simulink model "X1PFjicheng"  (R2024a)
settings: Solver=ode4  StartTime=0.0  StopTime=inf  FixedStep=0.05  RelTol=1e-3
values from neighbouring files (symbols this model uses):
  A0 = [app.A0XEditField.Value, app.A0YEditField.Value, app.A0ZEditField.Value]    [sendDubinsTCPData.m]    (also in sendLocalTCPData.m; sendTCPData.m)
  Delta = [app.Delta1EditField.Value,app.Delta2EditField.Value,app.Delta3EditField.Value,app.Delta4EditField.Value]    [sendDubinsTCPData.m]    (also in sendTCPData.m)
  down = app.downEditField.Value    [sendDubinsTCPData.m]    (also in sendTCPData.m)
  Kdelta = [app.Kdelta1EditField.Value,app.Kdelta2EditField.Value,app.Kdelta3EditField.Value,app.Kdelta4EditField.Value]    [sendDubinsTCPData.m]    (also in sendTCPData.m)
  P0 = [app.P0XEditField.Value, app.P0YEditField.Value, app.P0ZEditField.Value]    [sendDubinsTCPData.m]    (also in sendLocalTCPData.m; sendTCPData.m)
  Td = app.TdEditField.Value    [sendDubinsTCPData.m]    (also in sendTCPData.m)
  Tj = app.TjEditField.Value    [sendDubinsTCPData.m]    (also in sendTCPData.m)
  ud = app.udEditField.Value    [sendDubinsTCPData.m]    (also in sendTCPData.m)
  up = app.upEditField.Value    [sendDubinsTCPData.m]    (also in sendTCPData.m)
  Waypoints = evalin('base', 'Waypoints')    [planAUVPaths.m]    (also in planUAVPaths.m = csvread('CSV_waypoints.csv', 1, 0); sendTCPData.m = [app.Waypoints, column_of_z])
  WPNum = size(result_no_duplicates, 1)    [sendDubinsTCPData.m]    (also in sendLocalTCPData.m = size(waypoints, 1); sendTCPData.m = size(app.Waypoints, 1))
  z = app.ZEditField.Value    [sendDubinsTCPData.m]    (also in sendTCPData.m)
libraries: slpidlib x2
(part 1 of 2)
settings Model: Creator=22979  LastModifiedBy=22979
settings DataIOCC: SaveOperatingPoint=on  InspectSignalLogs=on  ReturnWorkspaceOutputs=off  LoggingFileName=losout.mat
settings DebuggingCC: AlgebraicLoopMsg=none  UnconnectedInputMsg=warning  UnconnectedOutputMsg=warning  UnconnectedLineMsg=warning
settings ModelReferenceCC: EnableRefExpFcnMdlSchedulingChecks=on
settings RTWCC: PackageGeneratedCodeAndArtifacts=on  GPUComputeCapability=3.5  DLArmComputeVersion=19.05

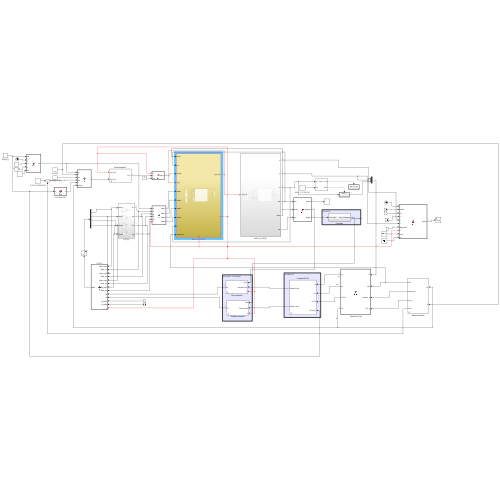
[thumbnail: Simulink's stored preview of the top-level diagram]
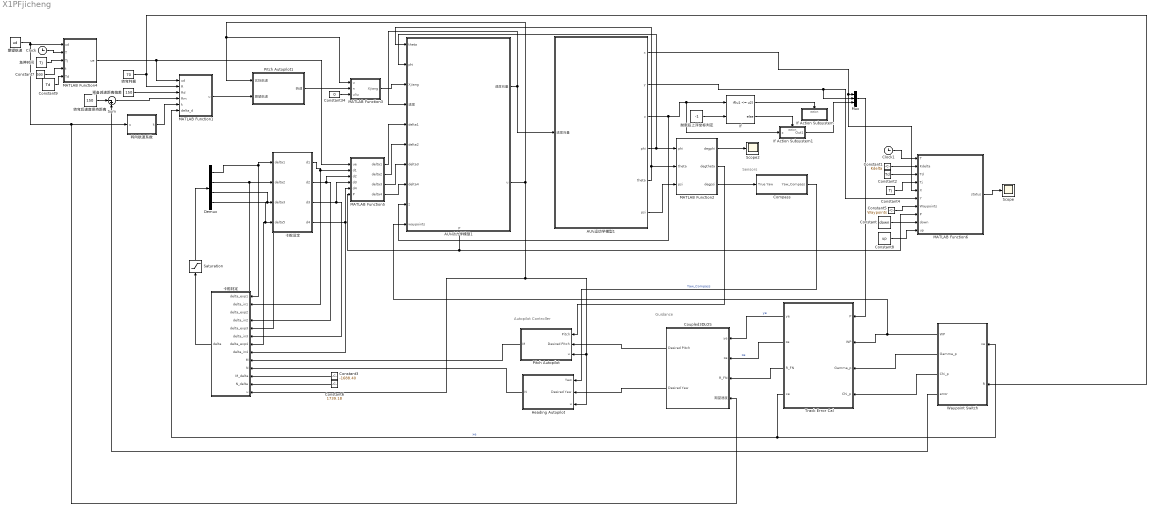
== system X1PFjicheng ==
  note: Sensors
  note: Guidance
  note: Autopilot Controller
  AUV动力学模型1 : Subsystem
      settings: PortSchema="{\"entries\":[{\"content\":{\"sides\":[{\"content\":{\"connectorIds\":[\"In1\",\"In2\",\"In3\",\"In4\",\"In5\",\"In6\",\"In7\",\"In8\",\"In9\",\"In10\"]},\"type\":\"ConnectorPlacement.EquallySpacedRectSide\",\"uuid\":\"1654708e-3081-4ea6-965b-5b7cd41b3ec5\"},{\"content\":{\"connectorIds\":[\"Out1\",\"Out2\"],\"side\":\"RIGHT\"},\"type\":\"ConnectorPlacement.EquallySpacedRectSide\",\"uuid\":\"9e07aa6c-7bc5-448a-bff9-c01bf6300cbd\"},{\"content\":{\"side\":\"TOP\"},\"type\":\"ConnectorPlacement.EquallySpacedRectSide\",\"uuid\":\"c074f735-85a1-4ba5-b9fb-1975a738e7a6\"},{\"content\":{\"connectorIds\":[\"Out3\"],\"side\":\"BOTTOM\"},\"type\":\"ConnectorPlacement.EquallySpacedRectSide\",\"uuid\":\"ec244679-bb4c-412e-b3fb-81b5c85a18e4\"}]},\"type\":\"ConnectorPlacement.EquallySpacedConnector\",\"uuid\":\"11f0b0be-650c-4135-b043-c000e16f372f\"}],\"packageUris\":[\"http://schema.mathworks.com/mf0/Connector/R2020b\"],\"version\":\"1.0\"}"
  AUV运动学模型1 : Subsystem
  Clock : Clock
  Clock1 : Clock
  Compass : Subsystem
  Constant : Constant  Value=down
  Constant1 : Constant  Value=Kdelta
  Constant2 : Constant  Value=Td
  Constant3 : Constant  Value=-1688.40
  Constant34 : Constant  Value=0
  Constant4 : Constant  Value=Tj
  Constant5 : Constant  Value=Waypoints
  Constant6 : Constant  Value=1739.18
  Constant7 : Constant  Value=500
  Constant8 : Constant  Value=up
  Constant9 : Constant  Value=Td
  Coupled3DLOS : Subsystem  mask{LOSAlg=LOS, Delta=26, Kapa=0.25, Gamma=0.3}
      mask prompts: LOSAlg "制导算法"; Delta "前视距离"; Kapa "漂角自适应估计增益"; Gamma "攻角自适应估计增益"
      mask TypeOptions LOSAlg: LOS | ALOS
      mask DialogControl DescGroupVar Prompt: 三维视线角制导
      mask DialogControl DescTextVar Prompt: 设置三维视线角制导参数：前视距离，漂角自适应估计增益，漂角自适应估计增益。自适应估计增益设置为0，屏蔽估计补偿；非0，启用估计补偿。
      mask DialogControl Container5 Prompt: 旋转制导算法
      mask DialogControl ParameterGroupVar Prompt: 设置制导参数
  Demux : Demux
  Heading Autopilot : Subsystem  mask{kp=1500, ki=0, kd=500}
      mask DialogControl DescGroupVar Prompt: Heading Autopilot
      mask DialogControl DescTextVar Prompt: 设置PID增益。
      mask DialogControl ParameterGroupVar Prompt: PID Parameter
  If : If  NumInputs=2  IfExpression=u1 <= u2
  If Action Subsystem : Subsystem  TreatAsAtomicUnit=on
  If Action Subsystem1 : Subsystem  TreatAsAtomicUnit=on
  MATLAB Function1 : MATLAB Function  TreatAsAtomicUnit=on
  MATLAB Function2 : MATLAB Function  TreatAsAtomicUnit=on
  MATLAB Function3 : MATLAB Function  TreatAsAtomicUnit=on
  MATLAB Function4 : MATLAB Function  TreatAsAtomicUnit=on
  MATLAB Function5 : MATLAB Function  TreatAsAtomicUnit=on
  MATLAB Function6 : MATLAB Function  TreatAsAtomicUnit=on
  Mux : Mux  Inputs=3
  Pitch Autopilot : Subsystem  mask{kp=2400, ki=0, kd=500}
      mask DialogControl DescGroupVar Prompt: Pitch Autopilot
      mask DialogControl DescTextVar Prompt: 设置PID控制增益。
      mask DialogControl ParameterGroupVar Prompt: PID Parameter
  Pitch Autopilot1 : Subsystem  mask{kp=600, ki=20, kd=0}
      mask DialogControl DescGroupVar Prompt: Pitch Autopilot
      mask DialogControl DescTextVar Prompt: 设置PID控制增益。
      mask DialogControl ParameterGroupVar Prompt: PID Parameter
  Saturation : Saturate  UpperLimit=0.4363  LowerLimit=-0.4363
  Scope : Scope
  Scope2 : Scope
  Sum : Sum  Inputs=|-+
  Track Error Cal : MATLAB Function  TreatAsAtomicUnit=on
  Waypoint Switch : Subsystem  mask{WP=Waypoints, WPNum=WPNum}
      mask prompts: WP "航点序列"; WPNum "航点个数"
      mask DialogControl DescGroupVar Prompt: 航点设置
      mask DialogControl DescTextVar Prompt: 设置航点序列和个数
  卡舵判定 : MATLAB Function  TreatAsAtomicUnit=on
  卡舵设定 : Subsystem
  急停时间 : Constant  Value=Tj
  抛载后上浮坐标判定 : Constant  Value=-1
  期望航速 : Constant  Value=ud
  转向航速系数 : MATLAB Function  TreatAsAtomicUnit=on
  转弯判据 : Constant  Value=70
  转弯后速度保持距离 : Constant  Value=150
  预备减速距离偏差 : Constant  Value=150
  wires:
  AUV运动学模型1/1(x) -> MATLAB Function6/5(X), Mux/1
  AUV运动学模型1/3(z) -> If/1, If Action Subsystem1/1(z), AUV动力学模型1/9(z)
  AUV运动学模型1/4(phi) -> MATLAB Function2/1(phi), AUV动力学模型1/2(phi)
  AUV运动学模型1/5(theta) -> AUV动力学模型1/1(theta), MATLAB Function2/2(theta)
  AUV运动学模型1/6(psi) -> MATLAB Function2/3(psi)
  AUV动力学模型1/1(速度向量) -> AUV动力学模型1/4(速度), AUV运动学模型1/1(速度向量)
  Track Error Cal/4(xe) -> Waypoint Switch/1(xe), MATLAB Function1/6(delta_d)  "xe"
  Waypoint Switch/3(Chi_p) -> Track Error Cal/4(Chi_p)
  Waypoint Switch/1(WP) -> AUV动力学模型1/10(waypoints), Track Error Cal/2(WP)
  Track Error Cal/2(ze) -> Coupled3DLOS/2(ze)  "ze"
  Track Error Cal/1(ye) -> Coupled3DLOS/1(ye)  "ye"
  Waypoint Switch/2(Gamma_p) -> Track Error Cal/3(Gamma_p)
  Track Error Cal/3(R_FN) -> Coupled3DLOS/3(R_FN)
  Coupled3DLOS/1(Desired Pitch) -> Pitch Autopilot/2(Desired Pitch)
  Coupled3DLOS/2(Desired Yaw) -> Heading Autopilot/2(Desired Yaw)
  Compass/1(Yaw_Compass) -> Heading Autopilot/1(Yaw)  "Yaw_Compass"
  MATLAB Function1/1(u) -> Pitch Autopilot1/2(期望航速)
  转弯后速度保持距离/1 -> Sum/1
  Pitch Autopilot1/1(转速) -> MATLAB Function3/2(n)
  Sum/1 -> MATLAB Function1/4(Rm)
  Constant34/1 -> MATLAB Function3/3(uliu)
  预备减速距离偏差/1 -> MATLAB Function1/3(Rd)
  转弯判据/1 -> Waypoint Switch/2(R), MATLAB Function1/2(R)
  AUV动力学模型1/2(u) -> Pitch Autopilot1/1(实际航速), MATLAB Function3/1(u), 卡舵判定/13(u), Pitch Autopilot/3(u), Heading Autopilot/3(u)
  Waypoint Switch/4(error) -> Sum/2
  AUV运动学模型1/2(y) -> Mux/2, MATLAB Function6/6(Y)
  Mux/1 -> Track Error Cal/1(P)
  MATLAB Function3/1(Xjiang) -> AUV动力学模型1/3(Xjiang)
  MATLAB Function2/2(degtheta) -> Pitch Autopilot/1(Pitch)
  MATLAB Function2/3(degpsi) -> Compass/1(True Yaw)
  Saturation/1 -> Demux/1
  MATLAB Function2/1(degphi) -> Scope2/1
  Demux/1 -> 卡舵判定/1(delta_exp1), 卡舵设定/1(delta1)
  卡舵设定/4(d4) -> MATLAB Function5/5(d4), 卡舵判定/8(delta_in4)
  Demux/2 -> 卡舵判定/3(delta_exp2), 卡舵设定/2(delta2)
  Demux/4 -> 卡舵设定/4(delta5), 卡舵判定/7(delta_exp4)
  Pitch Autopilot/1(M) -> 卡舵判定/9(M)
  Heading Autopilot/1(N) -> 卡舵判定/10(N)
  Constant3/1 -> 卡舵判定/11(M_delta)
  Constant6/1 -> 卡舵判定/12(N_delta)
  卡舵判定/1(delta) -> Saturation/1
  Demux/3 -> 卡舵判定/5(delta_exp3), 卡舵设定/3(delta3)
  卡舵设定/1(d1) -> 卡舵判定/2(delta_in1), MATLAB Function5/2(d1)
  卡舵设定/2(d2) -> MATLAB Function5/3(d2), 卡舵判定/4(delta_in2)
  卡舵设定/3(d3) -> MATLAB Function5/4(d3), 卡舵判定/6(delta_in3)
  抛载后上浮坐标判定/1 -> If/2
  If/1 -> If Action Subsystem/Action
  If/2 -> If Action Subsystem1/Action
  If Action Subsystem1/1(Out1) -> Mux/3
  Clock/1 -> MATLAB Function4/2(T)
  期望航速/1 -> Coupled3DLOS/4(期望速度), 转向航速系数/1(u), MATLAB Function4/1(ud)
  急停时间/1 -> MATLAB Function4/3(Tj)
  AUV动力学模型1/3(P) -> MATLAB Function5/6(P), MATLAB Function6/8(P)
  MATLAB Function5/1(delta1) -> AUV动力学模型1/5(delta1)
  MATLAB Function5/2(delta2) -> AUV动力学模型1/6(delta2)
  MATLAB Function5/3(delta3) -> AUV动力学模型1/7(delta3)
  MATLAB Function5/4(delta4) -> AUV动力学模型1/8(delta4)
  Constant1/1 -> MATLAB Function6/2(Kdelta)
  Constant2/1 -> MATLAB Function6/3(Td)
  Constant4/1 -> MATLAB Function6/4(Tj)
  MATLAB Function6/1(status) -> Scope/1
  Clock1/1 -> MATLAB Function6/1(T)
  Constant5/1 -> MATLAB Function6/7(Waypoints)
  Constant7/1 -> MATLAB Function4/4(t)
  MATLAB Function4/1(ue) -> MATLAB Function5/1(ue), MATLAB Function1/1(ud)
  转向航速系数/1(k) -> MATLAB Function1/5(k)
  Constant/1 -> MATLAB Function6/9(down)
  Constant8/1 -> MATLAB Function6/10(up)
  Constant9/1 -> MATLAB Function4/5(Td)

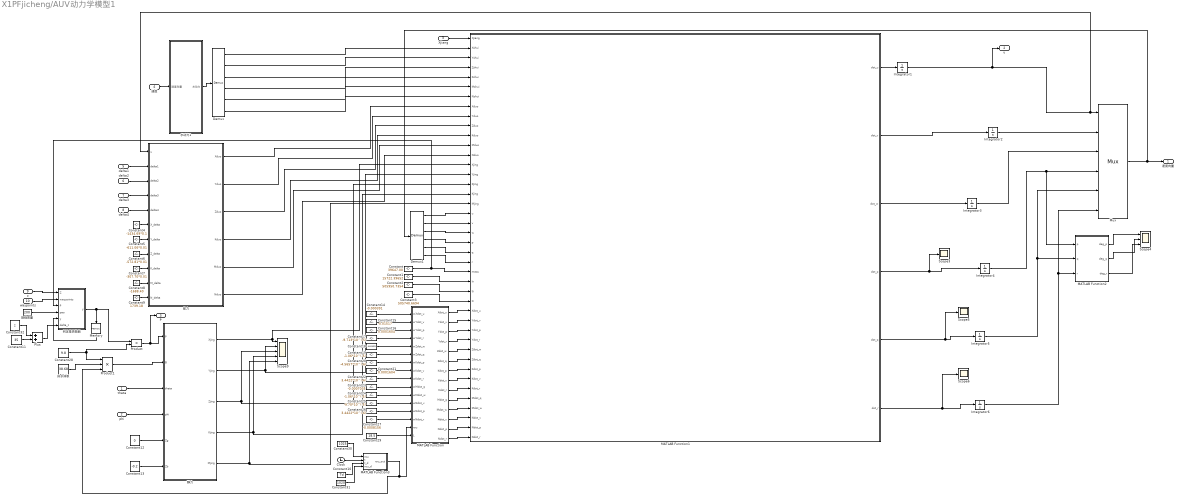
== system X1PFjicheng/AUV动力学模型1 ==
  theta : Inport
  phi : Inport  Port=2
  Xjiang : Inport  Port=3
  速度 : Inport  Port=4
  delta1 : Inport  Port=5
  delta2 : Inport  Port=6
  delta3 : Inport  Port=7
  delta4 : Inport  Port=8
  z : Inport  Port=9
  waypoints : Inport  Port=10
  Clock : Clock
  Constant : Constant  Value=39647.00
  Constant1 : Constant  Value=15722.39652
  Constant10 : Constant  Value=Td
  Constant11 : Constant  Value=35
  Constant12 : Constant  Value=0
  Constant13 : Constant  Value=-0.2
  Constant14 : Constant  Value=-0.000391
  Constant15 : Constant  Value=-0.01517
  Constant16 : Constant  Value=0.0001604
  Constant17 : Constant  Value=-9.713*10^(-5)
  Constant18 : Constant  Value=-0.0113
  Constant19 : Constant  Value=-1.06*10^(-5)
  Constant2 : Constant  Value=505950.7354
  Constant20 : Constant  Value=-4.5657*10^(-6)
  Constant21 : Constant  Value=0.0001604
  Constant22 : Constant  Value=3.4422*10^(-6)
  Constant23 : Constant  Value=-0.0007035
  Constant24 : Constant  Value=-1.06*10^(-5)
  Constant25 : Constant  Value=-9.70*10^(-5)
  Constant26 : Constant  Value=3.4422*10^(-6)
  Constant27 : Constant  Value=-0.0008156
  Constant28 : Constant  Value=9.8
  Constant29 : Constant  Value=18.5
  Constant3 : Constant  Value=505740.6694
  Constant30 : Constant  Value=1025
  Constant31 : Constant  Value=1020
  Constant32 : Constant  Value=z
  Constant4 : Constant  Value=-1434.69*0.1
  Constant5 : Constant  Value=-611.06*0.01
  Constant6 : Constant  Value=-572.81*0.01
  Constant7 : Constant  Value=-307.70*0.01
  Constant8 : Constant  Value=-1688.40
  Constant9 : Constant  Value=1739.18
  Demux : Demux  Outputs=6
  Demux1 : Demux  Outputs=6
  Integrator1 : Integrator  InitialCondition=0.01
  Integrator{2..6} (5 alike) : Integrator
  MATLAB Function : MATLAB Function  TreatAsAtomicUnit=on
  MATLAB Function1 : MATLAB Function  TreatAsAtomicUnit=on
  MATLAB Function2 : MATLAB Function  TreatAsAtomicUnit=on
  MATLAB Function3 : MATLAB Function  TreatAsAtomicUnit=on
  Memory : Memory
  Mux : Mux  Inputs=6
  Plus : Sum
  Product : Product
  Product1 : Product  Inputs=3
  Scope3 : Scope
  Scope4 : Scope  NumInputPorts=3
  Scope5 : Scope
  Scope6 : Scope
  Scope9 : Scope  NumInputPorts=5
  判定是否抛载 : MATLAB Function  TreatAsAtomicUnit=on
      settings: MinAlgLoopOccurrences=on
  抛载质量 : Constant  Value=200
  排水体积 : Constant  Value=38.68
  水动力1 : Subsystem
  舵力 : MATLAB Function  TreatAsAtomicUnit=on
  静力 : MATLAB Function  TreatAsAtomicUnit=on
  速度向量 : Outport
  u : Outport  Port=2
  P : Outport  Port=3
  wires:
  Integrator2/1 -> Mux/2
  Integrator5/1 -> MATLAB Function2/2(q), Mux/5
  Integrator3/1 -> Mux/3
  Integrator4/1 -> MATLAB Function2/1(p), Mux/4
  Integrator6/1 -> MATLAB Function2/3(r), Mux/6
  MATLAB Function1/3(dot_w) -> Integrator3/1
  MATLAB Function1/4(dot_p) -> Scope3/1, Integrator4/1
  MATLAB Function1/5(dot_q) -> Scope5/1, Integrator5/1
  MATLAB Function1/6(dot_r) -> Scope6/1, Integrator6/1
  MATLAB Function1/1(dot_u) -> Integrator1/1
  theta/1 -> 静力/3(theta)
  Mux/1 -> 速度向量/1, Demux1/1
  Demux/1 -> MATLAB Function1/2(Xshui)
  Demux/2 -> MATLAB Function1/3(Yshui)
  Demux/3 -> MATLAB Function1/4(Zshui)
  Demux/4 -> MATLAB Function1/5(Kshui)
  Demux/5 -> MATLAB Function1/6(Mshui)
  Demux/6 -> MATLAB Function1/7(Nshui)
  舵力/1(Xduo) -> MATLAB Function1/8(Xduo)
  舵力/2(Yduo) -> MATLAB Function1/9(Yduo)
  舵力/3(Zduo) -> MATLAB Function1/10(Zduo)
  舵力/4(Kduo) -> MATLAB Function1/11(Kduo)
  舵力/5(Mduo) -> MATLAB Function1/12(Mduo)
  舵力/6(Nduo) -> MATLAB Function1/13(Nduo)
  静力/1(Xjing) -> Scope9/1, MATLAB Function1/14(Xjing)
  静力/2(Yjing) -> MATLAB Function1/15(Yjing), Scope9/2
  静力/3(Zjing) -> MATLAB Function1/16(Zjing), Scope9/3
  静力/4(Kjing) -> MATLAB Function1/17(Kjing), Scope9/4
  静力/5(Mjing) -> MATLAB Function1/18(Mjing), Scope9/5
  Demux1/2 -> MATLAB Function1/20(v)
  Demux1/3 -> MATLAB Function1/21(w)
  Demux1/4 -> MATLAB Function1/22(p)
  Demux1/5 -> MATLAB Function1/23(q)
  Demux1/6 -> MATLAB Function1/24(r)
  Constant3/1 -> MATLAB Function1/28(Iz)
  Demux1/1 -> MATLAB Function1/19(u)
  Constant/1 -> 判定是否抛载/3(P), MATLAB Function1/25(mass)
  phi/1 -> 静力/4(phi)
  Constant12/1 -> 静力/5(Zg)
  Constant13/1 -> 静力/6(Zb)
  Constant2/1 -> MATLAB Function1/27(Iy)
  Constant1/1 -> MATLAB Function1/26(Ix)
  Constant14/1 -> MATLAB Function/1(wXdot_u)
  MATLAB Function/1(Xdot_u) -> MATLAB Function1/29(Xdot_u)
  MATLAB Function/2(Ydot_v) -> MATLAB Function1/30(Ydot_v)
  MATLAB Function/3(Ydot_p) -> MATLAB Function1/31(Ydot_p)
  MATLAB Function/4(Ydot_r) -> MATLAB Function1/32(Ydot_r)
  MATLAB Function/5(Zdot_w) -> MATLAB Function1/33(Zdot_w)
  MATLAB Function/6(Zdot_q) -> MATLAB Function1/34(Zdot_q)
  MATLAB Function/7(Kdot_p) -> MATLAB Function1/35(Kdot_p)
  MATLAB Function/8(Kdot_v) -> MATLAB Function1/36(Kdot_v)
  MATLAB Function/9(Kdot_r) -> MATLAB Function1/37(Kdot_r)
  MATLAB Function/10(Mdot_q) -> MATLAB Function1/38(Mdot_q)
  MATLAB Function/11(Mdot_w) -> MATLAB Function1/39(Mdot_w)
  MATLAB Function/12(Ndot_v) -> MATLAB Function1/40(Ndot_v)
  MATLAB Function/13(Ndot_p) -> MATLAB Function1/41(Ndot_p)
  MATLAB Function/14(Ndot_r) -> MATLAB Function1/42(Ndot_r)
  Constant15/1 -> MATLAB Function/2(wYdot_v)
  Constant16/1 -> MATLAB Function/3(wYdot_p)
  Constant17/1 -> MATLAB Function/4(wYdot_r)
  Constant18/1 -> MATLAB Function/5(wZdot_w)
  Constant19/1 -> MATLAB Function/6(wZdot_q)
  Constant20/1 -> MATLAB Function/7(wKdot_p)
  Constant21/1 -> MATLAB Function/8(wKdot_v)
  Constant22/1 -> MATLAB Function/9(wKdot_r)
  Constant23/1 -> MATLAB Function/10(wMdot_q)
  Constant24/1 -> MATLAB Function/11(wMdot_w)
  Constant25/1 -> MATLAB Function/12(wNdot_v)
  Constant26/1 -> MATLAB Function/13(wNdot_p)
  Constant27/1 -> MATLAB Function/14(wNdot_r)
  Constant29/1 -> MATLAB Function/16(L)
  Integrator1/1 -> u/1, Mux/1, 舵力/1(u)
  MATLAB Function1/2(dot_v) -> Integrator2/1
  MATLAB Function2/1(deg_p) -> Scope4/1
  MATLAB Function2/2(deg_q) -> Scope4/2
  MATLAB Function2/3(deg_r) -> Scope4/3
  Constant4/1 -> 舵力/6(X_delta)
  Constant6/1 -> 舵力/8(Z_delta)
  Constant7/1 -> 舵力/9(K_delta)
  Constant8/1 -> 舵力/10(M_delta)
  Constant9/1 -> 舵力/11(N_delta)
  Constant5/1 -> 舵力/7(Y_delta)
  水动力1/1(水动力) -> Demux/1
  速度/1 -> 水动力1/1(速度向量)
  Xjiang/1 -> MATLAB Function1/1(Xjiang)
  Clock/1 -> MATLAB Function3/2(t)
  Constant30/1 -> MATLAB Function3/1(rou)
  MATLAB Function3/1(rou_out) -> Product1/3, MATLAB Function/15(rou)
  排水体积/1 -> Product1/2
  Constant28/1 -> Product/2, Product1/1
  Product1/1 -> 静力/2(B)
  Constant31/1 -> MATLAB Function3/4(rou_d)
  Constant10/1 -> MATLAB Function3/3(t_d)
  抛载质量/1 -> 判定是否抛载/4(pao)
  waypoints/1 -> 判定是否抛载/2(waypoints)
  z/1 -> 判定是否抛载/1(Z)
  Product/1 -> P/1, 静力/1(P)
  判定是否抛载/1(y) -> Memory/1, Product/1
  Memory/1 -> 判定是否抛载/5("y ")
  delta1/1 -> 舵力/2(delta1)
  delta2/1 -> 舵力/3(delta2)
  delta3/1 -> 舵力/4(delta3)
  delta4/1 -> 舵力/5(delta4)
  Constant11/1 -> Plus/2
  Plus/1 -> 判定是否抛载/6(delta_z)
  Constant32/1 -> Plus/1

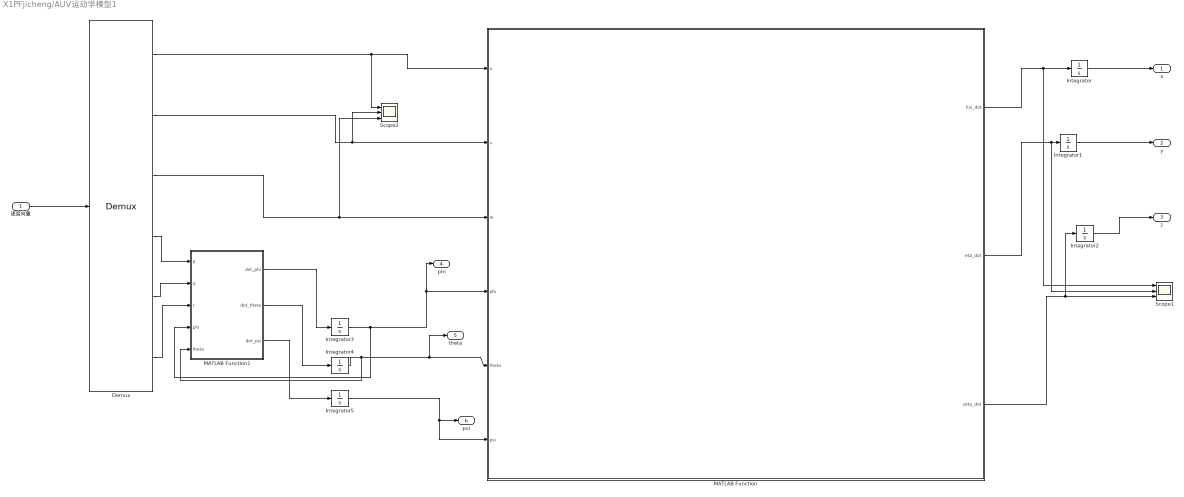
== system X1PFjicheng/AUV运动学模型1 ==
  速度向量 : Inport
  Demux : Demux  Outputs=6
  Integrator : Integrator  InitialCondition=P0(1)
  Integrator1 : Integrator  InitialCondition=P0(2)
  Integrator2 : Integrator  InitialCondition=P0(3)
  Integrator3 : Integrator  InitialCondition=A0(1)*pi/180
  Integrator4 : Integrator  InitialCondition=A0(2)*pi/180
  Integrator5 : Integrator  InitialCondition=A0(3)*pi/180
  MATLAB Function : MATLAB Function  TreatAsAtomicUnit=on
  MATLAB Function1 : MATLAB Function  TreatAsAtomicUnit=on
  Scope1 : Scope  NumInputPorts=3
  Scope2 : Scope  NumInputPorts=3
  x : Outport
  y : Outport  Port=2
  z : Outport  Port=3
  phi : Outport  Port=4
  theta : Outport  Port=5
  psi : Outport  Port=6
  wires:
  Integrator2/1 -> z/1
  Integrator1/1 -> y/1
  MATLAB Function/2(eta_dot) -> Scope1/2, Integrator1/1
  MATLAB Function/1(ksi_dot) -> Integrator/1, Scope1/1
  MATLAB Function/3(zeta_dot) -> Integrator2/1, Scope1/3
  Demux/1 -> Scope2/1, MATLAB Function/1(u)
  Demux/2 -> Scope2/2, MATLAB Function/2(v)
  Demux/3 -> Scope2/3, MATLAB Function/3(w)
  速度向量/1 -> Demux/1
  Integrator3/1 -> MATLAB Function1/4(phi), MATLAB Function/4(phi), phi/1
  Integrator4/1 -> MATLAB Function1/5(theta), theta/1, MATLAB Function/5(theta)
  Integrator5/1 -> MATLAB Function/6(psi), psi/1
  Demux/5 -> MATLAB Function1/2(q)
  Demux/4 -> MATLAB Function1/1(p)
  Demux/6 -> MATLAB Function1/3(r)
  MATLAB Function1/1(dot_phi) -> Integrator3/1
  MATLAB Function1/2(dot_theta) -> Integrator4/1
  MATLAB Function1/3(dot_psi) -> Integrator5/1
  Integrator/1 -> x/1

== system X1PFjicheng/Compass ==
  True Yaw : Inport
  Add : Sum
  Add1 : Sum
  Add2 : Sum
  Constant : Constant  Value=round(rand*20-10)
  Constant1 : Constant  Value=0
  Gain : Gain  Gain=0
  Integrator : Integrator
  MATLAB Function : MATLAB Function  TreatAsAtomicUnit=on
  Random Number : RandomNumber  Commented=on  Variance=0.05  Seed=round(rand*20)  SampleTime=1
  Yaw_Compass : Outport
  wires:
  Constant/1 -> Add1/2  "bias"
  Integrator/1 -> Add1/1, Gain/1  "noise"
  Gain/1 -> Add/2
  Add/1 -> Integrator/1
  Add1/1 -> Add2/1  "Compass_Noise"
  True Yaw/1 -> Add2/2
  MATLAB Function/1(u) -> Yaw_Compass/1
  Add2/1 -> MATLAB Function/1(in)
  Constant1/1 -> Add/1

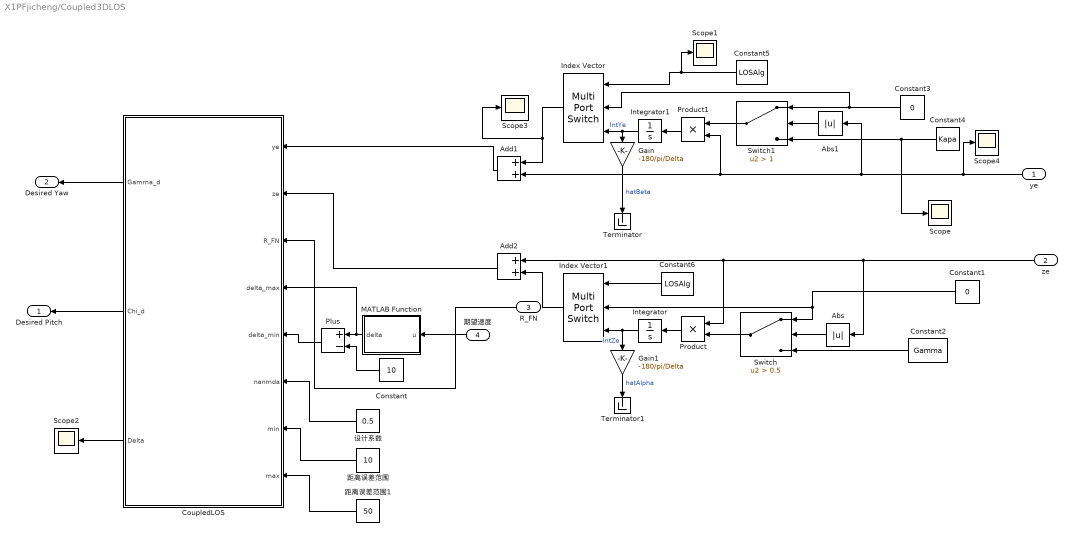
== system X1PFjicheng/Coupled3DLOS ==
  ye : Inport
  ze : Inport  Port=2
  R_FN : Inport  Port=3
  期望速度 : Inport  Port=4
  Abs : Abs  SaturateOnIntegerOverflow=off
  Abs1 : Abs  SaturateOnIntegerOverflow=off
  Add1 : Sum
  Add2 : Sum
  Constant : Constant  Value=10
  Constant1 : Constant  Value=0
  Constant2 : Constant  Value=Gamma
  Constant3 : Constant  Value=0
  Constant4 : Constant  Value=Kapa
  Constant5 : Constant  Value=LOSAlg
  Constant6 : Constant  Value=LOSAlg
  CoupledLOS : MATLAB Function  TreatAsAtomicUnit=on
  Gain : Gain  Gain=-180/pi/Delta
  Gain1 : Gain  Gain=-180/pi/Delta
  Index Vector : MultiPortSwitch  Inputs=2  SaturateOnIntegerOverflow=off  InputSameDT=off
  Index Vector1 : MultiPortSwitch  Inputs=2  SaturateOnIntegerOverflow=off  InputSameDT=off
  Integrator : Integrator
  Integrator1 : Integrator
  MATLAB Function : MATLAB Function  TreatAsAtomicUnit=on
  Plus : Sum  Inputs=+-
  Product : Product
  Product1 : Product
  Scope{,1..4} (5 alike) : Scope
  Switch : Switch  Criteria=u2 > Threshold  Threshold=0.5  SaturateOnIntegerOverflow=off  InputSameDT=off
  Switch1 : Switch  Criteria=u2 > Threshold  Threshold=1  SaturateOnIntegerOverflow=off  InputSameDT=off
  Terminator : Terminator
  Terminator1 : Terminator
  设计系数 : Constant  Value=0.5
  距离误差范围 : Constant  Value=10
  距离误差范围1 : Constant  Value=50
  Desired Pitch : Outport
  Desired Yaw : Outport  Port=2
  wires:
  Abs1/1 -> Switch1/2
  ze/1 -> Abs/1, Add2/1, Product/1
  Constant2/1 -> Switch/3
  Abs/1 -> Switch/2
  Product/1 -> Integrator/1
  Constant4/1 -> Scope/1, Switch1/3
  Constant1/1 -> Index Vector1/2, Switch/1
  ye/1 -> Add1/2, Product1/2, Abs1/1, Scope4/1
  Integrator/1 -> Gain1/1, Index Vector1/3  "IntZe"
  Add2/1 -> CoupledLOS/2(ze)
  Product1/1 -> Integrator1/1
  Switch/1 -> Product/2
  CoupledLOS/2(Chi_d) -> Desired Pitch/1
  Switch1/1 -> Product1/1
  Constant3/1 -> Index Vector/2, Switch1/1
  Add1/1 -> CoupledLOS/1(ye)
  CoupledLOS/1(Gamma_d) -> Desired Yaw/1
  Integrator1/1 -> Gain/1, Index Vector/3  "IntYe"
  R_FN/1 -> CoupledLOS/3(R_FN)
  Constant5/1 -> Scope1/1, Index Vector/1
  Index Vector/1 -> Add1/1, Scope3/1
  Constant6/1 -> Index Vector1/1
  Index Vector1/1 -> Add2/2
  Gain/1 -> Terminator/1  "hatBeta"
  Gain1/1 -> Terminator1/1  "hatAlpha"
  MATLAB Function/1(delta) -> CoupledLOS/4(delta_max), Plus/1
  设计系数/1 -> CoupledLOS/6(nanmda)
  距离误差范围/1 -> CoupledLOS/7(min)
  距离误差范围1/1 -> CoupledLOS/8(max)
  CoupledLOS/3(Delta) -> Scope2/1
  期望速度/1 -> MATLAB Function/1(u)
  Plus/1 -> CoupledLOS/5(delta_min)
  Constant/1 -> Plus/2

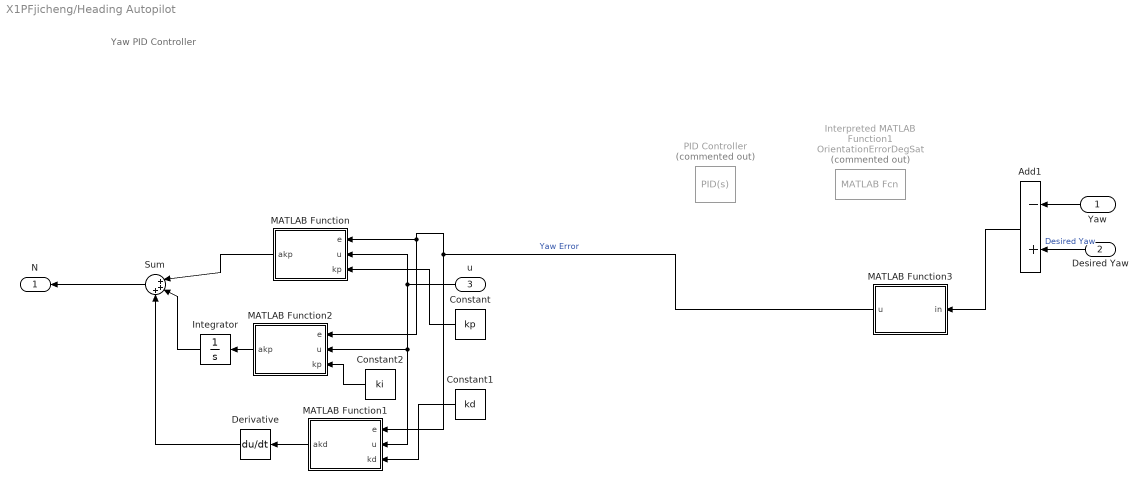
== system X1PFjicheng/Heading Autopilot ==
  note: Yaw PID Controller
  Yaw : Inport
  Desired Yaw : Inport  Port=2
  u : Inport  Port=3
  Add1 : Sum  Inputs=-+
  Constant : Constant  Value=kp
  Constant1 : Constant  Value=kd
  Constant2 : Constant  Value=ki
  Derivative : Derivative
  Integrator : Integrator
  Interpreted MATLAB Function1 : MATLABFcn  Commented=on  MATLABFcn=OrientationErrorDegSat  OutputDimensions=1
  MATLAB Function : MATLAB Function  TreatAsAtomicUnit=on
  MATLAB Function1 : MATLAB Function  TreatAsAtomicUnit=on
  MATLAB Function2 : MATLAB Function  TreatAsAtomicUnit=on
  MATLAB Function3 : MATLAB Function  TreatAsAtomicUnit=on
  PID Controller : slpidlib/PID Controller  Commented=on  Controller=PID  Form=Parallel  TimeDomain=Continuous-time  UseExternalTs=off  SampleTime=-1  IntegratorMethod=Forward Euler  FilterMethod=Forward Euler  ControllerParametersSource=internal  P=kp  I=ki  UseKiTs=off  D=kd  UseExternalDerivativeSource=off  N=100  UseFilter=on  TunerSelectOption=Transfer Function Based (PID Tuner App)  InitialConditionSource=internal  InitialConditionForIntegrator=0  InitialConditionForFilter=0  DifferentiatorICPrevScaledInput=0  ExternalReset=none  TrackingMode=off  Kt=1  LimitOutput=off  SatLimitsSource=internal  UpperSaturationLimit=inf  LowerSaturationLimit=-inf  LinearizeAsGain=on  AntiWindupMode=none  Kb=1  LimitIntegrator=off  UpperIntegratorSaturationLimit=inf  LowerIntegratorSaturationLimit=-inf  POutMin=[]  POutMax=[]  IOutMin=[]  IOutMax=[]  DOutMin=[]  DOutMax=[]  NOutMin=[]  NOutMax=[]  SumOutMin=[]  SumOutMax=[]  SaturationOutMin=[]  SaturationOutMax=[]  PParamMin=[]  PParamMax=[]  IParamMin=[]  IParamMax=[]  DParamMin=[]  DParamMax=[]  NParamMin=[]  NParamMax=[]  KbParamMin=[]  KbParamMax=[]  KtParamMin=[]  KtParamMax=[]  KbOutMin=[]  KbOutMax=[]  KtOutMin=[]  KtOutMax=[]  IntegratorOutMin=[]  IntegratorOutMax=[]  FilterOutMin=[]  FilterOutMax=[]  SumI1OutMin=[]  SumI1OutMax=[]  SumI2OutMin=[]  SumI2OutMax=[]  SumI3OutMin=[]  SumI3OutMax=[]  SumI4OutMin=[]  SumI4OutMax=[]  SumDOutMin=[]  SumDOutMax=[]  DifferentiatorOutMin=[]  DifferentiatorOutMax=[]  FilterDiffOutCoefMin=[]  FilterDiffOutCoefMax=[]  ReciprocalOutMin=[]  ReciprocalOutMax=[]  SumDenOutMin=[]  SumDenOutMax=[]  SumNumOutMin=[]  SumNumOutMax=[]  DivideOutMin=[]  DivideOutMax=[]  UdiffTsProdOutMin=[]  UdiffTsProdOutMax=[]  NTsProdOutMin=[]  NTsProdOutMax=[]  UintegralTsProdOutMin=[]  UintegralTsProdOutMax=[]  UngainTsProdOutMin=[]  UngainTsProdOutMax=[]  ClampingZeroOutDataTypeStr=Inherit: Inherit via back propagation  ClampingZeroOutMin=[]  ClampingZeroOutMax=[]  FilterDenConstantOutDataTypeStr=Inherit: Inherit via back propagation  FilterDenConstantOutMin=[]  FilterDenConstantOutMax=[]  PCopyOutDataTypeStr=Inherit: Inherit via back propagation  PCopyOutMin=[]  PCopyOutMax=[]  NCopyOutDataTypeStr=Inherit: Inherit via back propagation  NCopyOutMin=[]  NCopyOutMax=[]  IntegratorContinuousStateAttributes=''  IntegratorStateMustResolveToSignalObject=off  IntegratorRTWStateStorageClass=Auto  FilterContinuousStateAttributes=''  FilterStateMustResolveToSignalObject=off  FilterRTWStateStorageClass=Auto  ParallelPVariant=InternalParameters  IdealPVariant=Disabled  IVariant=InternalParameters  DVariant=InternalParameters  IntegratorVariant=Continuous  SatVariant=Disabled  AWVariant=Passthrough  PCopyVariant=Disabled  TRVariant=Disabled  FdbkBlocksVariant=Forward  IdealPFdbkVariant=Disabled  SatFdbkVariant=Disabled  DerivativeFilterVariant=ContFilter  NVariant=InternalParameters  NCopyVariant=Disabled  FilterICVariant=InternalICsFilter  IntegratorICVariant=InternalICs  ExternalResetVariant=Disabled  TRSumVariant=Passthrough  SumFdbkVariant=Disabled  SumVariant=Sum_PID  TsampFilterVariant=InternalTs  TsampNgainVariant=Passthrough  TsampIntegralVariant=Disabled_SignalSpec  ExternalSaturationOutDataTypeStr=Inherit: Same as second input  DerivativeSourceVariant=ErrorSignal
  Sum : Sum  Inputs=|+++
  N : Outport
  wires:
  Yaw/1 -> Add1/1
  Add1/1 -> MATLAB Function3/1(in)
  Desired Yaw/1 -> Add1/2  "Desired Yaw"
  Constant1/1 -> MATLAB Function1/3(kd)
  MATLAB Function1/1(akd) -> Derivative/1
  Constant/1 -> MATLAB Function/3(kp)
  u/1 -> MATLAB Function1/2(u), MATLAB Function2/2(u), MATLAB Function/2(u)
  Constant2/1 -> MATLAB Function2/3(kp)
  MATLAB Function2/1(akp) -> Integrator/1
  MATLAB Function/1(akp) -> Sum/1
  Integrator/1 -> Sum/2
  Derivative/1 -> Sum/3
  Sum/1 -> N/1
  MATLAB Function3/1(u) -> MATLAB Function2/1(e), MATLAB Function/1(e), MATLAB Function1/1(e)  "Yaw Error"

== system X1PFjicheng/If Action Subsystem ==
  Action Port : ActionPort  ActionPortLabel=if(u1 <= u2)
  Constant : Constant
  Stop Simulation : Stop
  wires:
  Constant/1 -> Stop Simulation/1

== system X1PFjicheng/If Action Subsystem1 ==
  z : Inport
  Action Port : ActionPort  ActionPortLabel=else
  Out1 : Outport
  wires:
  z/1 -> Out1/1

== system X1PFjicheng/Pitch Autopilot ==
  note: Pitch PID Controller
  Pitch : Inport
  Desired Pitch : Inport  Port=2
  u : Inport  Port=3
  Add1 : Sum  Inputs=-+
  Constant : Constant  Value=kp
  Constant1 : Constant  Value=kd
  Constant2 : Constant  Value=ki
  Derivative : Derivative
  Integrator : Integrator
  MATLAB Function : MATLAB Function  TreatAsAtomicUnit=on
  MATLAB Function1 : MATLAB Function  TreatAsAtomicUnit=on
  MATLAB Function2 : MATLAB Function  TreatAsAtomicUnit=on
  Saturation : Saturate  UpperLimit=25  LowerLimit=-25
  Sum : Sum  Inputs=|+++
  M : Outport
  wires:
  Desired Pitch/1 -> Saturation/1
  Pitch/1 -> Add1/1
  Saturation/1 -> Add1/2  "Desired Pitch"
  Sum/1 -> M/1
  MATLAB Function/1(akp) -> Sum/1
  Constant/1 -> MATLAB Function/3(kp)
  Add1/1 -> MATLAB Function/1(e), MATLAB Function2/1(e), MATLAB Function1/1(e)
  Constant1/1 -> MATLAB Function1/3(kd)
  MATLAB Function1/1(akd) -> Derivative/1
  Derivative/1 -> Sum/2
  u/1 -> MATLAB Function2/2(u), MATLAB Function/2(u), MATLAB Function1/2(u)
  Constant2/1 -> MATLAB Function2/3(ki)
  MATLAB Function2/1(akp) -> Integrator/1
  Integrator/1 -> Sum/3

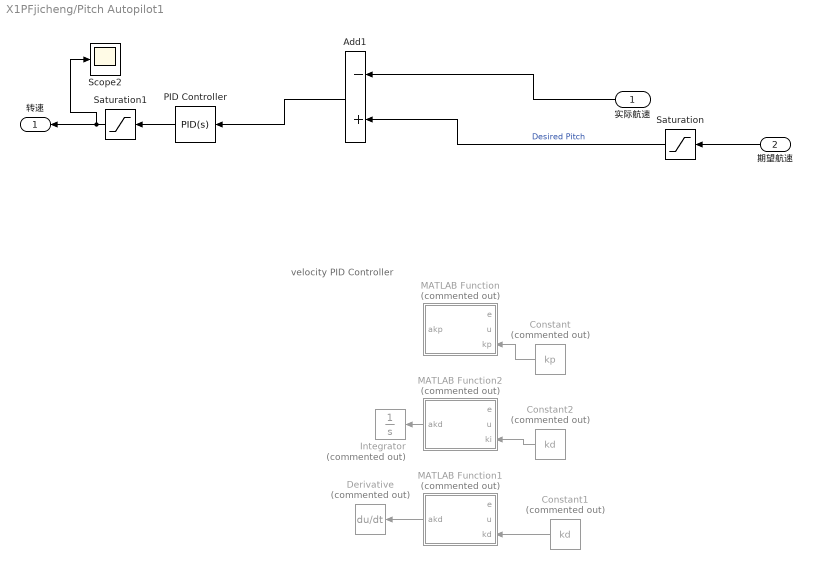
== system X1PFjicheng/Pitch Autopilot1 ==
  note: velocity PID Controller
  实际航速 : Inport
  期望航速 : Inport  Port=2
  Add1 : Sum  Inputs=-+
  Constant : Constant  Commented=on  Value=kp
  Constant1 : Constant  Commented=on  Value=kd
  Constant2 : Constant  Commented=on  Value=kd
  Derivative : Derivative  Commented=on
  Integrator : Integrator  Commented=on
  MATLAB Function : MATLAB Function  Commented=on  TreatAsAtomicUnit=on
  MATLAB Function1 : MATLAB Function  Commented=on  TreatAsAtomicUnit=on
  MATLAB Function2 : MATLAB Function  Commented=on  TreatAsAtomicUnit=on
  PID Controller : slpidlib/PID Controller  Controller=PID  Form=Parallel  TimeDomain=Continuous-time  UseExternalTs=off  SampleTime=-1  IntegratorMethod=Forward Euler  FilterMethod=Forward Euler  ControllerParametersSource=internal  P=kp  I=ki  UseKiTs=off  D=kd  UseExternalDerivativeSource=off  N=100  UseFilter=on  TunerSelectOption=Transfer Function Based (PID Tuner App)  InitialConditionSource=internal  InitialConditionForIntegrator=0  InitialConditionForFilter=0  DifferentiatorICPrevScaledInput=0  ExternalReset=none  TrackingMode=off  Kt=1  LimitOutput=off  SatLimitsSource=internal  UpperSaturationLimit=inf  LowerSaturationLimit=-inf  LinearizeAsGain=on  AntiWindupMode=none  Kb=1  LimitIntegrator=off  UpperIntegratorSaturationLimit=inf  LowerIntegratorSaturationLimit=-inf  POutMin=[]  POutMax=[]  IOutMin=[]  IOutMax=[]  DOutMin=[]  DOutMax=[]  NOutMin=[]  NOutMax=[]  SumOutMin=[]  SumOutMax=[]  SaturationOutMin=[]  SaturationOutMax=[]  PParamMin=[]  PParamMax=[]  IParamMin=[]  IParamMax=[]  DParamMin=[]  DParamMax=[]  NParamMin=[]  NParamMax=[]  KbParamMin=[]  KbParamMax=[]  KtParamMin=[]  KtParamMax=[]  KbOutMin=[]  KbOutMax=[]  KtOutMin=[]  KtOutMax=[]  IntegratorOutMin=[]  IntegratorOutMax=[]  FilterOutMin=[]  FilterOutMax=[]  SumI1OutMin=[]  SumI1OutMax=[]  SumI2OutMin=[]  SumI2OutMax=[]  SumI3OutMin=[]  SumI3OutMax=[]  SumI4OutMin=[]  SumI4OutMax=[]  SumDOutMin=[]  SumDOutMax=[]  DifferentiatorOutMin=[]  DifferentiatorOutMax=[]  FilterDiffOutCoefMin=[]  FilterDiffOutCoefMax=[]  ReciprocalOutMin=[]  ReciprocalOutMax=[]  SumDenOutMin=[]  SumDenOutMax=[]  SumNumOutMin=[]  SumNumOutMax=[]  DivideOutMin=[]  DivideOutMax=[]  UdiffTsProdOutMin=[]  UdiffTsProdOutMax=[]  NTsProdOutMin=[]  NTsProdOutMax=[]  UintegralTsProdOutMin=[]  UintegralTsProdOutMax=[]  UngainTsProdOutMin=[]  UngainTsProdOutMax=[]  ClampingZeroOutDataTypeStr=Inherit: Inherit via back propagation  ClampingZeroOutMin=[]  ClampingZeroOutMax=[]  FilterDenConstantOutDataTypeStr=Inherit: Inherit via back propagation  FilterDenConstantOutMin=[]  FilterDenConstantOutMax=[]  PCopyOutDataTypeStr=Inherit: Inherit via back propagation  PCopyOutMin=[]  PCopyOutMax=[]  NCopyOutDataTypeStr=Inherit: Inherit via back propagation  NCopyOutMin=[]  NCopyOutMax=[]  IntegratorContinuousStateAttributes=''  IntegratorStateMustResolveToSignalObject=off  IntegratorRTWStateStorageClass=Auto  FilterContinuousStateAttributes=''  FilterStateMustResolveToSignalObject=off  FilterRTWStateStorageClass=Auto  ParallelPVariant=InternalParameters  IdealPVariant=Disabled  IVariant=InternalParameters  DVariant=InternalParameters  IntegratorVariant=Continuous  SatVariant=Disabled  AWVariant=Passthrough  PCopyVariant=Disabled  TRVariant=Disabled  FdbkBlocksVariant=Forward  IdealPFdbkVariant=Disabled  SatFdbkVariant=Disabled  DerivativeFilterVariant=ContFilter  NVariant=InternalParameters  NCopyVariant=Disabled  FilterICVariant=InternalICsFilter  IntegratorICVariant=InternalICs  ExternalResetVariant=Disabled  TRSumVariant=Passthrough  SumFdbkVariant=Disabled  SumVariant=Sum_PID  TsampFilterVariant=InternalTs  TsampNgainVariant=Passthrough  TsampIntegralVariant=Disabled_SignalSpec  ExternalSaturationOutDataTypeStr=Inherit: Same as second input  DerivativeSourceVariant=ErrorSignal
  Saturation : Saturate  UpperLimit=7.8  LowerLimit=0
  Saturation1 : Saturate  UpperLimit=450  LowerLimit=0
  Scope2 : Scope
  转速 : Outport
  wires:
  期望航速/1 -> Saturation/1
  Saturation/1 -> Add1/2  "Desired Pitch"
  MATLAB Function1/1(akd) -> Derivative/1
  Constant/1 -> MATLAB Function/3(kp)
  Constant1/1 -> MATLAB Function1/3(kd)
  Saturation1/1 -> Scope2/1, 转速/1
  MATLAB Function2/1(akd) -> Integrator/1
  Constant2/1 -> MATLAB Function2/3(ki)
  实际航速/1 -> Add1/1
  Add1/1 -> PID Controller/1
  PID Controller/1 -> Saturation1/1

== system X1PFjicheng/Waypoint Switch ==
  xe : Inport
  R : Inport  Port=2
  Constant2 : Constant  Value=WPNum+1
  Constant3 : Constant
  If : If  NumInputs=2  IfExpression=u1 >= u2
  If Action Subsystem : Subsystem  TreatAsAtomicUnit=on
  If Action Subsystem1 : Subsystem  TreatAsAtomicUnit=on
  Memory : Memory  InitialCondition=1  InheritSampleTime=on
  Memory1 : Memory  InitialCondition=5  InheritSampleTime=on
  Sum : Sum  Inputs=|++
  Sum1 : Sum  Inputs=|+-
  Triggered Subsystem : Subsystem  TreatAsAtomicUnit=on
  WP : Outport
  Gamma_p : Outport  Port=2
  Chi_p : Outport  Port=3
  error : Outport  Port=4
  wires:
  Constant2/1 -> If/2
  If Action Subsystem1/2(Gamma_p) -> Gamma_p/1
  Sum1/1 -> Memory1/1
  Memory/1 -> Sum/1
  If/2 -> If Action Subsystem1/Action
  xe/1 -> Sum1/1
  Sum/1 -> Triggered Subsystem/1(In1)
  Constant3/1 -> Sum/2
  If Action Subsystem1/1(WP_(n+1)) -> WP/1
  Triggered Subsystem/1(WPID) -> If/1, If Action Subsystem1/1(WPID), Memory/1  "WPID"
  R/1 -> Sum1/2
  If/1 -> If Action Subsystem/Action
  Memory1/1 -> Triggered Subsystem/Trigger
  If Action Subsystem1/3(Chi_p) -> Chi_p/1
  If Action Subsystem1/4(error) -> error/1

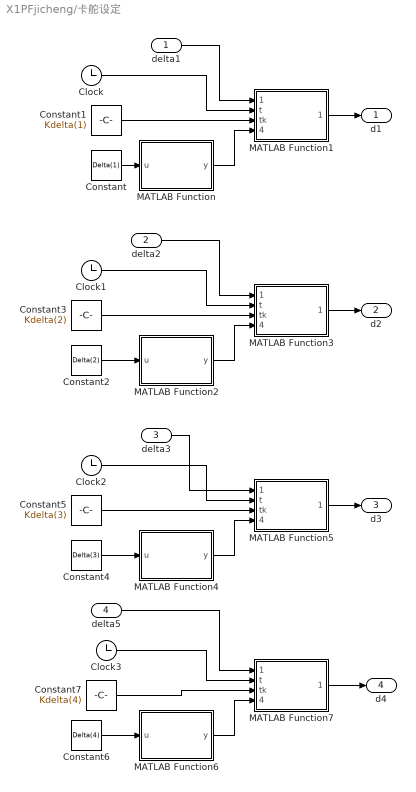
== system X1PFjicheng/卡舵设定 ==
  delta1 : Inport
  delta2 : Inport  Port=2
  delta3 : Inport  Port=3
  delta5 : Inport  Port=4
  Clock{,1..3} (4 alike) : Clock
  Constant : Constant  Value=Delta(1)
  Constant1 : Constant  Value=Kdelta(1)
  Constant2 : Constant  Value=Delta(2)
  Constant3 : Constant  Value=Kdelta(2)
  Constant4 : Constant  Value=Delta(3)
  Constant5 : Constant  Value=Kdelta(3)
  Constant6 : Constant  Value=Delta(4)
  Constant7 : Constant  Value=Kdelta(4)
  MATLAB Function : MATLAB Function  TreatAsAtomicUnit=on
  MATLAB Function1 : MATLAB Function  TreatAsAtomicUnit=on
  MATLAB Function2 : MATLAB Function  TreatAsAtomicUnit=on
  MATLAB Function3 : MATLAB Function  TreatAsAtomicUnit=on
  MATLAB Function4 : MATLAB Function  TreatAsAtomicUnit=on
  MATLAB Function5 : MATLAB Function  TreatAsAtomicUnit=on
  MATLAB Function6 : MATLAB Function  TreatAsAtomicUnit=on
  MATLAB Function7 : MATLAB Function  TreatAsAtomicUnit=on
  d1 : Outport
  d2 : Outport  Port=2
  d3 : Outport  Port=3
  d4 : Outport  Port=4
  wires:
  Constant/1 -> MATLAB Function/1(u)
  delta1/1 -> MATLAB Function1/1(delta_in)
  Clock/1 -> MATLAB Function1/2(t)
  MATLAB Function1/1(delta_out) -> d1/1
  Constant1/1 -> MATLAB Function1/3(tk)
  MATLAB Function/1(y) -> MATLAB Function1/4(delta_k)
  Clock1/1 -> MATLAB Function3/2(t)
  MATLAB Function3/1(delta_out) -> d2/1
  Constant2/1 -> MATLAB Function2/1(u)
  delta2/1 -> MATLAB Function3/1(delta_in)
  MATLAB Function2/1(y) -> MATLAB Function3/4(delta_k)
  Constant3/1 -> MATLAB Function3/3(tk)
  Constant5/1 -> MATLAB Function5/3(tk)
  delta3/1 -> MATLAB Function5/1(delta_in)
  Clock2/1 -> MATLAB Function5/2(t)
  MATLAB Function5/1(delta_out) -> d3/1
  MATLAB Function4/1(y) -> MATLAB Function5/4(delta_k)
  Constant4/1 -> MATLAB Function4/1(u)
  MATLAB Function6/1(y) -> MATLAB Function7/4(delta_k)
  Constant7/1 -> MATLAB Function7/3(tk)
  Constant6/1 -> MATLAB Function6/1(u)
  MATLAB Function7/1(delta_out) -> d4/1
  delta5/1 -> MATLAB Function7/1(delta_in)
  Clock3/1 -> MATLAB Function7/2(t)

== system X1PFjicheng/AUV动力学模型1/水动力1 ==
  note: N水动力系数
  速度向量 : Inport
  Constant : Constant  Value=1025
  Constant1 : Constant  Value=18.5
  Demux : Demux  Outputs=6
  K水动力系数 : Subsystem
  MATLAB Function : MATLAB Function  TreatAsAtomicUnit=on
  Mux : Mux  Inputs=6
  M水动力系数 : Subsystem
  Scope : Scope  NumInputPorts=6
  Scope2 : Scope
  Scope7 : Scope
  Subsystem5 : Subsystem
  X水动力系数 : Subsystem
  Y水动力系数 : Subsystem
  Z水动力系数 : Subsystem
  水动力 : Outport
  wires:
  MATLAB Function/1(Xshui) -> Scope/1, Mux/1
  Demux/1 -> Scope7/1, MATLAB Function/73(u)
  Demux/2 -> MATLAB Function/74(v)
  Demux/3 -> Scope2/1, MATLAB Function/75(w)
  Demux/4 -> MATLAB Function/76(p)
  Demux/5 -> MATLAB Function/77(q)
  Demux/6 -> MATLAB Function/78(r)
  速度向量/1 -> Demux/1
  MATLAB Function/2(Yshui) -> Mux/2, Scope/2
  MATLAB Function/3(Zshui) -> Mux/3, Scope/3
  MATLAB Function/4(Kshui) -> Scope/4, Mux/4
  MATLAB Function/5(Mshui) -> Scope/5, Mux/5
  MATLAB Function/6(Nshui) -> Scope/6, Mux/6
  Mux/1 -> 水动力/1
  X水动力系数/1(Xqq) -> MATLAB Function/1(Xqq)
  X水动力系数/2(Xrr) -> MATLAB Function/2(Xrr)
  X水动力系数/3(Xrp) -> MATLAB Function/3(Xrp)
  X水动力系数/4(Xvr) -> MATLAB Function/4(Xvr)
  X水动力系数/5(Xwq) -> MATLAB Function/5(Xwq)
  X水动力系数/6(Xuu) -> MATLAB Function/6(Xuu)
  X水动力系数/7(Xvv) -> MATLAB Function/7(Xvv)
  X水动力系数/8(Xww) -> MATLAB Function/8(Xww)
  Y水动力系数/1(Yp_p) -> MATLAB Function/9(Yp_p)
  Y水动力系数/2(Ypq) -> MATLAB Function/10(Ypq)
  Y水动力系数/3(Yqr) -> MATLAB Function/11(Yqr)
  Y水动力系数/4(Yvq) -> MATLAB Function/12(Yvq)
  Y水动力系数/5(Ywp) -> MATLAB Function/13(Ywp)
  Y水动力系数/6(Ywr) -> MATLAB Function/14(Ywr)
  Y水动力系数/7(Yr) -> MATLAB Function/15(Yr)
  Y水动力系数/8(Yp) -> MATLAB Function/16(Yp)
  Y水动力系数/9(Yv_r) -> MATLAB Function/17(Yv_r)
  Y水动力系数/10(Y0) -> MATLAB Function/18(Y0)
  Y水动力系数/11(Yv) -> MATLAB Function/19(Yv)
  Y水动力系数/12(Yv-v) -> MATLAB Function/20(Yv_v)
  Y水动力系数/13(Yvw) -> MATLAB Function/21(Yvw)
  Z水动力系数/1(Zpp) -> MATLAB Function/22(Zpp)
  Z水动力系数/2(Zrr) -> MATLAB Function/23(Zrr)
  Z水动力系数/3(Zrp) -> MATLAB Function/24(Zrp)
  Z水动力系数/4(Zvr) -> MATLAB Function/25(Zvr)
  Z水动力系数/5(Zvp) -> MATLAB Function/26(Zvp)
  Z水动力系数/6(Zq) -> MATLAB Function/27(Zq)
  Z水动力系数/7(Zw_q) -> MATLAB Function/28(Zw_q)
  Z水动力系数/8(Z0) -> MATLAB Function/29(Z0)
  Z水动力系数/9(Zw) -> MATLAB Function/30(Zw)
  Z水动力系数/10(Zw_w) -> MATLAB Function/31(Zw_w)
  Z水动力系数/11(Z-w) -> MATLAB Function/32(Z_w)
  Z水动力系数/12(Zww) -> MATLAB Function/33(Zww)
  K水动力系数/1(Kqr) -> MATLAB Function/34(Kqr)
  K水动力系数/2(Kpq) -> MATLAB Function/35(Kpq)
  K水动力系数/3(Kp_p) -> MATLAB Function/36(Kp_p)
  K水动力系数/4(Kp) -> MATLAB Function/37(Kp)
  K水动力系数/5(Kr) -> MATLAB Function/38(Kr)
  K水动力系数/6(Kvq) -> MATLAB Function/39(Kvq)
  K水动力系数/7(Kwp) -> MATLAB Function/40(Kwp)
  K水动力系数/8(Kwr) -> MATLAB Function/41(Kwr)
  K水动力系数/9(K0) -> MATLAB Function/42(K0)
  K水动力系数/10(Kv) -> MATLAB Function/43(Kv)
  K水动力系数/11(Kv_v) -> MATLAB Function/44(Kv_v)
  K水动力系数/12(Kvw) -> MATLAB Function/45(Kvw)
  M水动力系数/1(Mpp) -> MATLAB Function/46(Mpp)
  M水动力系数/2(Mrr) -> MATLAB Function/47(Mrr)
  M水动力系数/3(Mrp) -> MATLAB Function/48(Mrp)
  M水动力系数/4(Mq_q) -> MATLAB Function/49(Mq_q)
  M水动力系数/5(Mvr) -> MATLAB Function/50(Mvr)
  M水动力系数/6(Mvp) -> MATLAB Function/51(Mvp)
  M水动力系数/7(Mq) -> MATLAB Function/52(Mq)
  M水动力系数/8(M_wq) -> MATLAB Function/53(M_wq)
  M水动力系数/9(M0) -> MATLAB Function/54(M0)
  M水动力系数/10(Mw) -> MATLAB Function/55(Mw)
  M水动力系数/11(Mw_w) -> MATLAB Function/56(Mw_w)
  M水动力系数/12(M_w) -> MATLAB Function/57(M_w)
  M水动力系数/13(Mww) -> MATLAB Function/58(Mww)
  M水动力系数/14(Mvv) -> MATLAB Function/59(Mvv)
  Subsystem5/1(Npq) -> MATLAB Function/60(Npq)
  Subsystem5/2(Nqr) -> MATLAB Function/61(Nqr)
  Subsystem5/3(Nr_r) -> MATLAB Function/62(Nr_r)
  Subsystem5/4(Nwr) -> MATLAB Function/63(Nwr)
  Subsystem5/5(Nwp) -> MATLAB Function/64(Nwp)
  Subsystem5/6(Nvq) -> MATLAB Function/65(Nvq)
  Subsystem5/7(Np) -> MATLAB Function/66(Np)
  Subsystem5/8(Nr) -> MATLAB Function/67(Nr)
  Subsystem5/9(N_vr) -> MATLAB Function/68(N_vr)
  Subsystem5/10(N0) -> MATLAB Function/69(N0)
  Subsystem5/11(Nv) -> MATLAB Function/70(Nv)
  Subsystem5/12(Nv_v) -> MATLAB Function/71(Nv_v)
  Subsystem5/13(Nvw) -> MATLAB Function/72(Nvw)
  Constant1/1 -> MATLAB Function/80(L)
  Constant/1 -> MATLAB Function/79(rou)

== system X1PFjicheng/Waypoint Switch/If Action Subsystem ==
  Action Port : ActionPort  ActionPortLabel=if(u1 >= u2)
  Constant : Constant
  Stop Simulation : Stop
  wires:
  Constant/1 -> Stop Simulation/1

== system X1PFjicheng/Waypoint Switch/If Action Subsystem1 ==
  WPID : Inport
  Action Port : ActionPort  ActionPortLabel=else
  Constant1 : Constant  Value=P0
  Constant2 : Constant  Value=WP
  MATLAB Function1 : MATLAB Function  TreatAsAtomicUnit=on
  WP_(n+1) : Outport
  Gamma_p : Outport  Port=2
  Chi_p : Outport  Port=3
  error : Outport  Port=4
  wires:
  MATLAB Function1/2(Gamma_p) -> Gamma_p/1  "Gamma_p"
  MATLAB Function1/1(WP) -> WP_(n+1)/1
  Constant2/1 -> MATLAB Function1/1(WPSEQ)
  WPID/1 -> MATLAB Function1/2(WPID)  "WPID"
  MATLAB Function1/3(Chi_p) -> Chi_p/1  "Chi_p"
  Constant1/1 -> MATLAB Function1/3(P0)
  MATLAB Function1/4(error) -> error/1

== system X1PFjicheng/Waypoint Switch/Triggered Subsystem ==
  In1 : Inport
  Trigger : TriggerPort  TriggerType=falling  VariantControl=Variant
  WPID : Outport  InitialOutput=1
  wires:
  In1/1 -> WPID/1

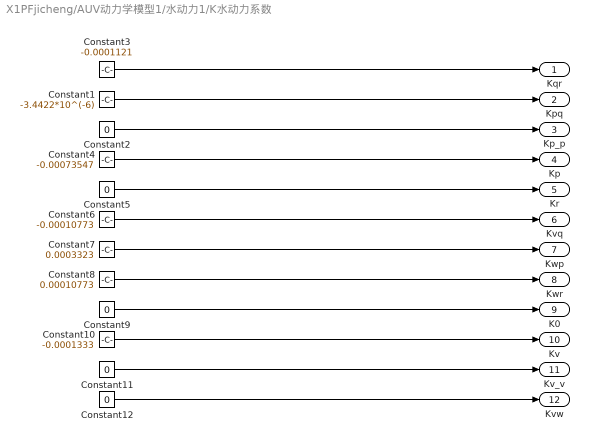
== system X1PFjicheng/AUV动力学模型1/水动力1/K水动力系数 ==
  Constant1 : Constant  Value=-3.4422*10^(-6)
  Constant10 : Constant  Value=-0.0001333
  Constant{2,5,9,11..12} (5 alike) : Constant  Value=0
  Constant3 : Constant  Value=-0.0001121
  Constant4 : Constant  Value=-0.00073547
  Constant6 : Constant  Value=-0.00010773
  Constant7 : Constant  Value=0.0003323
  Constant8 : Constant  Value=0.00010773
  Kqr : Outport
  Kpq : Outport  Port=2
  Kp_p : Outport  Port=3
  Kp : Outport  Port=4
  Kr : Outport  Port=5
  Kvq : Outport  Port=6
  Kwp : Outport  Port=7
  Kwr : Outport  Port=8
  K0 : Outport  Port=9
  Kv : Outport  Port=10
  Kv_v : Outport  Port=11
  Kvw : Outport  Port=12
  wires:
  Constant7/1 -> Kwp/1
  Constant6/1 -> Kvq/1
  Constant2/1 -> Kp_p/1
  Constant1/1 -> Kpq/1
  Constant11/1 -> Kv_v/1
  Constant5/1 -> Kr/1
  Constant9/1 -> K0/1
  Constant4/1 -> Kp/1
  Constant3/1 -> Kqr/1
  Constant8/1 -> Kwr/1
  Constant12/1 -> Kvw/1
  Constant10/1 -> Kv/1

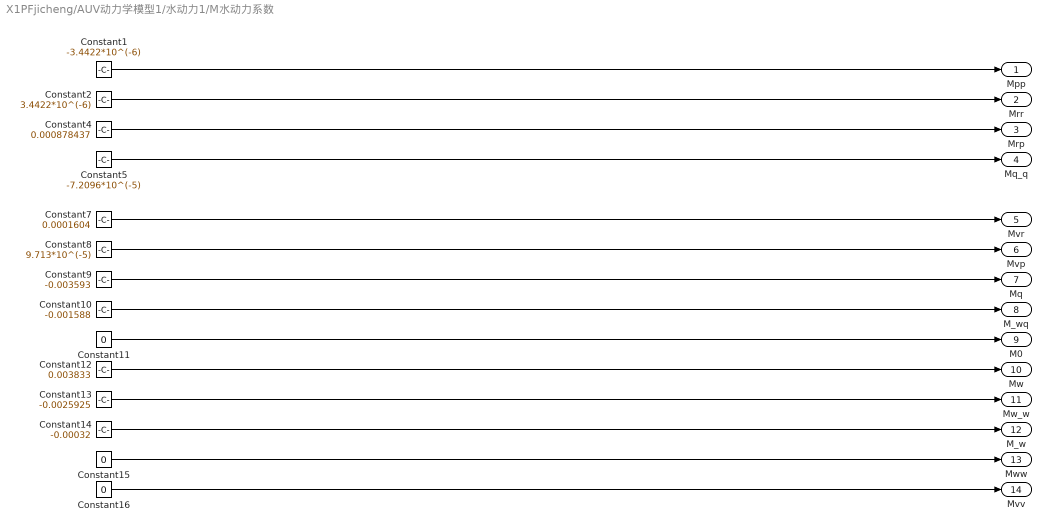
== system X1PFjicheng/AUV动力学模型1/水动力1/M水动力系数 ==
  Constant1 : Constant  Value=-3.4422*10^(-6)
  Constant10 : Constant  Value=-0.001588
  Constant11 : Constant  Value=0
  Constant12 : Constant  Value=0.003833
  Constant13 : Constant  Value=-0.0025925
  Constant14 : Constant  Value=-0.00032
  Constant15 : Constant  Value=0
  Constant16 : Constant  Value=0
  Constant2 : Constant  Value=3.4422*10^(-6)
  Constant4 : Constant  Value=0.000878437
  Constant5 : Constant  Value=-7.2096*10^(-5)
  Constant7 : Constant  Value=0.0001604
  Constant8 : Constant  Value=9.713*10^(-5)
  Constant9 : Constant  Value=-0.003593
  Mpp : Outport
  Mrr : Outport  Port=2
  Mrp : Outport  Port=3
  Mq_q : Outport  Port=4
  Mvr : Outport  Port=5
  Mvp : Outport  Port=6
  Mq : Outport  Port=7
  M_wq : Outport  Port=8
  M0 : Outport  Port=9
  Mw : Outport  Port=10
  Mw_w : Outport  Port=11
  M_w : Outport  Port=12
  Mww : Outport  Port=13
  Mvv : Outport  Port=14
  wires:
  Constant1/1 -> Mpp/1
  Constant4/1 -> Mrp/1
  Constant2/1 -> Mrr/1
  Constant8/1 -> Mvp/1
  Constant7/1 -> Mvr/1
  Constant16/1 -> Mvv/1
  Constant15/1 -> Mww/1
  Constant14/1 -> M_w/1
  Constant10/1 -> M_wq/1
  Constant13/1 -> Mw_w/1
  Constant12/1 -> Mw/1
  Constant5/1 -> Mq_q/1
  Constant9/1 -> Mq/1
  Constant11/1 -> M0/1

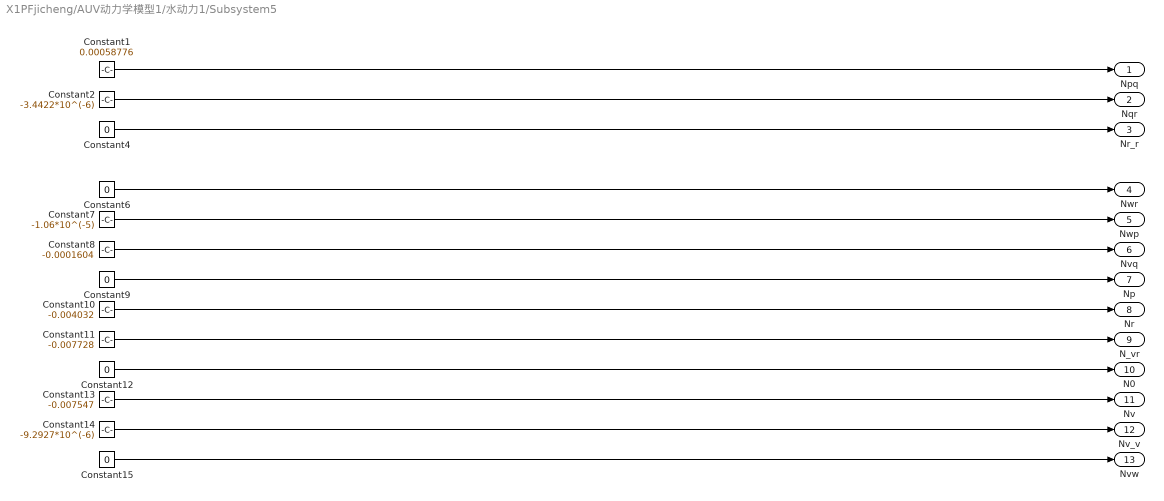
== system X1PFjicheng/AUV动力学模型1/水动力1/Subsystem5 ==
  Constant1 : Constant  Value=0.00058776
  Constant10 : Constant  Value=-0.004032
  Constant11 : Constant  Value=-0.007728
  Constant{4,6,9,12,15} (5 alike) : Constant  Value=0
  Constant13 : Constant  Value=-0.007547
  Constant14 : Constant  Value=-9.2927*10^(-6)
  Constant2 : Constant  Value=-3.4422*10^(-6)
  Constant7 : Constant  Value=-1.06*10^(-5)
  Constant8 : Constant  Value=-0.0001604
  Npq : Outport
  Nqr : Outport  Port=2
  Nr_r : Outport  Port=3
  Nwr : Outport  Port=4
  Nwp : Outport  Port=5
  Nvq : Outport  Port=6
  Np : Outport  Port=7
  Nr : Outport  Port=8
  N_vr : Outport  Port=9
  N0 : Outport  Port=10
  Nv : Outport  Port=11
  Nv_v : Outport  Port=12
  Nvw : Outport  Port=13
  wires:
  Constant1/1 -> Npq/1
  Constant15/1 -> Nvw/1
  Constant7/1 -> Nwp/1
  Constant9/1 -> Np/1
  Constant10/1 -> Nr/1
  Constant6/1 -> Nwr/1
  Constant12/1 -> N0/1
  Constant8/1 -> Nvq/1
  Constant2/1 -> Nqr/1
  Constant4/1 -> Nr_r/1
  Constant11/1 -> N_vr/1
  Constant14/1 -> Nv_v/1
  Constant13/1 -> Nv/1

== system X1PFjicheng/AUV动力学模型1/水动力1/X水动力系数 ==
  Constant : Constant  Value=-1.06*10^(-5)
  Constant1 : Constant  Value=9.713*10^(-5)
  Constant2 : Constant  Value=-0.0001604
  Constant4 : Constant  Value=-0.00196583
  Constant5 : Constant  Value=0.008986
  Constant6 : Constant  Value=-0.000918711
  Constant7 : Constant  Value=0
  Constant8 : Constant  Value=0
  Xqq : Outport
  Xrr : Outport  Port=2
  Xrp : Outport  Port=3
  Xvr : Outport  Port=4
  Xwq : Outport  Port=5
  Xuu : Outport  Port=6
  Xvv : Outport  Port=7
  Xww : Outport  Port=8
  wires:
  Constant1/1 -> Xrr/1
  Constant6/1 -> Xuu/1
  Constant/1 -> Xqq/1
  Constant2/1 -> Xrp/1
  Constant8/1 -> Xww/1
  Constant5/1 -> Xwq/1
  Constant4/1 -> Xvr/1
  Constant7/1 -> Xvv/1

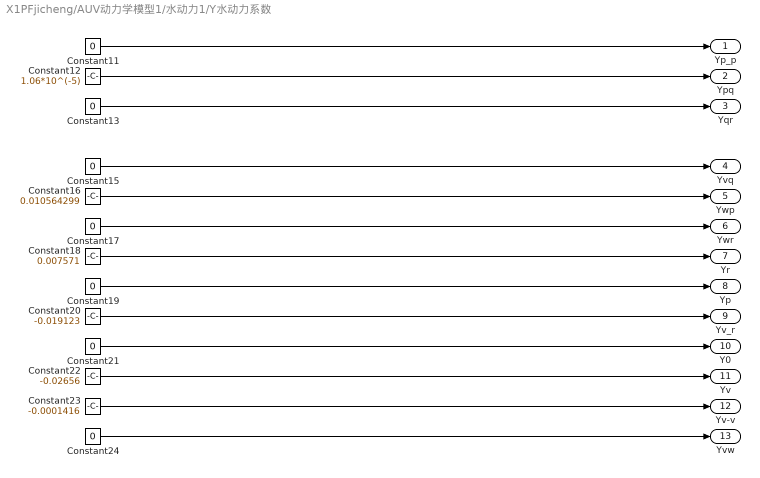
== system X1PFjicheng/AUV动力学模型1/水动力1/Y水动力系数 ==
  Constant{11,13,15,17,19,21,24} (7 alike) : Constant  Value=0
  Constant12 : Constant  Value=1.06*10^(-5)
  Constant16 : Constant  Value=0.010564299
  Constant18 : Constant  Value=0.007571
  Constant20 : Constant  Value=-0.019123
  Constant22 : Constant  Value=-0.02656
  Constant23 : Constant  Value=-0.0001416
  Yp_p : Outport
  Ypq : Outport  Port=2
  Yqr : Outport  Port=3
  Yvq : Outport  Port=4
  Ywp : Outport  Port=5
  Ywr : Outport  Port=6
  Yr : Outport  Port=7
  Yp : Outport  Port=8
  Yv_r : Outport  Port=9
  Y0 : Outport  Port=10
  Yv : Outport  Port=11
  Yv-v : Outport  Port=12
  Yvw : Outport  Port=13
  wires:
  Constant20/1 -> Yv_r/1
  Constant15/1 -> Yvq/1
  Constant13/1 -> Yqr/1
  Constant24/1 -> Yvw/1
  Constant18/1 -> Yr/1
  Constant19/1 -> Yp/1
  Constant17/1 -> Ywr/1
  Constant22/1 -> Yv/1
  Constant11/1 -> Yp_p/1
  Constant21/1 -> Y0/1
  Constant16/1 -> Ywp/1
  Constant23/1 -> Yv-v/1
  Constant12/1 -> Ypq/1

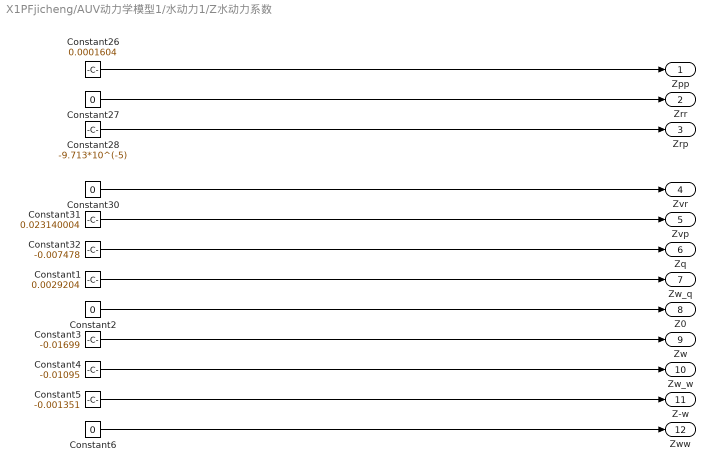
== system X1PFjicheng/AUV动力学模型1/水动力1/Z水动力系数 ==
  Constant1 : Constant  Value=0.0029204
  Constant{2,6,27,30} (4 alike) : Constant  Value=0
  Constant26 : Constant  Value=0.0001604
  Constant28 : Constant  Value=-9.713*10^(-5)
  Constant3 : Constant  Value=-0.01699
  Constant31 : Constant  Value=0.023140004
  Constant32 : Constant  Value=-0.007478
  Constant4 : Constant  Value=-0.01095
  Constant5 : Constant  Value=-0.001351
  Zpp : Outport
  Zrr : Outport  Port=2
  Zrp : Outport  Port=3
  Zvr : Outport  Port=4
  Zvp : Outport  Port=5
  Zq : Outport  Port=6
  Zw_q : Outport  Port=7
  Z0 : Outport  Port=8
  Zw : Outport  Port=9
  Zw_w : Outport  Port=10
  Z-w : Outport  Port=11
  Zww : Outport  Port=12
  wires:
  Constant5/1 -> Z-w/1
  Constant4/1 -> Zw_w/1
  Constant28/1 -> Zrp/1
  Constant6/1 -> Zww/1
  Constant32/1 -> Zq/1
  Constant27/1 -> Zrr/1
  Constant26/1 -> Zpp/1
  Constant31/1 -> Zvp/1
  Constant3/1 -> Zw/1
  Constant1/1 -> Zw_q/1
  Constant30/1 -> Zvr/1
  Constant2/1 -> Z0/1

== matlab function X1PFjicheng/AUV运动学模型1/MATLAB Function1 ==
  data: p input; q input; r input; phi input; dot_phi output; dot_theta output; dot_psi output; theta input
function [dot_phi,dot_theta,dot_psi] = qupdt(p,q,r,phi,theta)
dot_phi=p+q*tan(theta)*sin(phi)+r*tan(theta)*cos(phi);
dot_theta=q*cos(phi)-r*sin(phi);
dot_psi=(q*sin(phi)+r*cos(phi))/cos(theta);

== matlab function X1PFjicheng/AUV动力学模型1/MATLAB Function ==
  data: wXdot_u input; Xdot_u output; Ydot_v output; Ydot_p output; Ydot_r output; Zdot_w output; Zdot_q output; wYdot_v input; wYdot_p input; wYdot_r input; wZdot_w input; wZdot_q input; wKdot_p input; wKdot_v input; wKdot_r input; wMdot_q input; wMdot_w input; wNdot_v input; wNdot_p input; wNdot_r input; rou input; L input; Kdot_p output; Kdot_v output; Kdot_r output; Mdot_q output; Mdot_w output; Ndot_v output; Ndot_p output; Ndot_r output
function [Xdot_u,Ydot_v,Ydot_p,Ydot_r,Zdot_w,Zdot_q, Kdot_p,Kdot_v,Kdot_r,Mdot_q,Mdot_w,Ndot_v,Ndot_p,Ndot_r]  = fcn(wXdot_u,wYdot_v,wYdot_p,wYdot_r,wZdot_w,wZdot_q, wKdot_p,wKdot_v,wKdot_r,wMdot_q,wMdot_w,wNdot_v,wNdot_p,wNdot_r,rou,L)
Xdot_u=0.5*rou*L^3*wXdot_u;
Ydot_v=0.5*rou*L^3*wYdot_v;
Ydot_p=0.5*rou*L^4*wYdot_p;
Ydot_r=0.5*rou*L^4*wYdot_r;
Zdot_w=0.5*rou*L^3*wZdot_w;
Zdot_q=0.5*rou*L^4*wZdot_q;
Kdot_p=0.5*rou*L^5*wKdot_p;
Kdot_v=0.5*rou*L^4*wKdot_v;
Kdot_r=0.5*rou*L^5*wKdot_r;
Mdot_q=0.5*rou*L^5*wMdot_q;
Mdot_w=0.5*rou*L^4*wMdot_w;
Ndot_v=0.5*rou*L^4*wNdot_v;
Ndot_p=0.5*rou*L^5*wNdot_p;
Ndot_r=0.5*rou*L^5*wNdot_r;

== matlab function X1PFjicheng/MATLAB Function2 ==
  data: phi input; degphi output; theta input; psi input; degtheta output; degpsi output
function [degphi,degtheta,degpsi]= fcn(phi,theta,psi)
degphi=rad2deg(phi);
degtheta=rad2deg(theta);
degpsi=rad2deg(psi);
